simulink model "hinfinity"  (R2016a)
settings: Solver=VariableStepAuto  StartTime=0.0  StopTime=10.0  RelTol=1e-3
libraries: cstblocks x3
settings Model: Creator=engrh  LastModifiedBy=engrh
settings OptimizationCC: DefaultParameterBehavior=Inlined  BufferReuse=off
settings DebuggingCC: InitInArrayFormatMsg=none

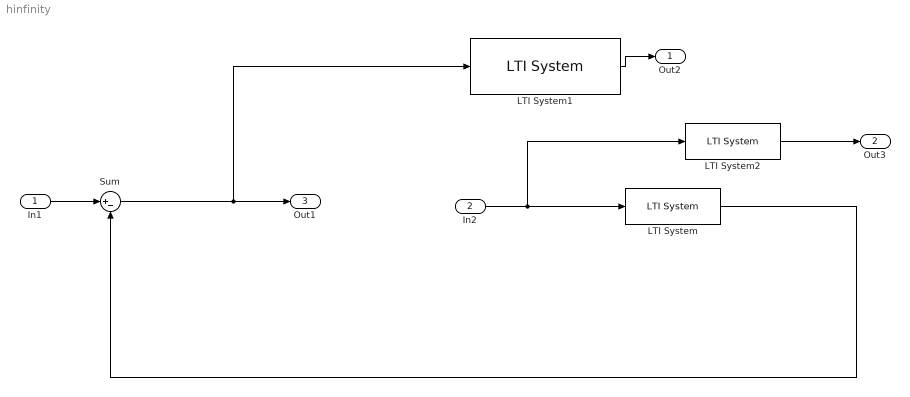
== system hinfinity ==
  In1 : Inport
  In2 : Inport  Port=2  PortDimensions=2
  LTI System : cstblocks/LTI System  sys=G  IC=[]
  LTI System1 : cstblocks/LTI System  sys=Ws  IC=[]
  LTI System2 : cstblocks/LTI System  sys=Wu  IC=[]
  Sum : Sum  Inputs=|+-
  Out2 : Outport
  Out3 : Outport  Port=2
  Out1 : Outport  Port=3  PortDimensions=2
  wires:
  In1/1 -> Sum/1
  In2/1 -> LTI System2/1, LTI System/1
  Sum/1 -> LTI System1/1, Out1/1
  LTI System/1 -> Sum/2
  LTI System1/1 -> Out2/1
  LTI System2/1 -> Out3/1
